simulink model "Evaluate_positioning_control_action"  (R2016b)
settings: Solver=ode1  StartTime=0.0  StopTime=pre_time  FixedStep=T_sample  MinStep=1e-4  RelTol=1e-3
undefined symbols (not defined in the file): A_f, Activator, B_f, C_f, D_f, filter_initial_condition, Integral_action, out_int, pre_time, x_0, x_start
libraries: qbmove_library x2, QB_pacer_lib x1
settings Model: Creator=Franco  LastModifiedBy=Franco
settings DataIOCC: LimitDataPoints=on  SaveFormat=Array  SignalLoggingSaveFormat=ModelDataLogs
settings OptimizationCC: ExpressionDepthLimit=2147483647  EfficientMapNaN2IntZero=off  LifeSpan=inf
settings DebuggingCC: UnderspecifiedInitializationDetection=Classic  MergeDetectMultiDrivingBlocksExec=none  SolverPrmCheckMsg=warning  FcnCallInpInsideContextMsg=warning  AllowSymbolicDim=off  StateNameClashWarn=warning  SFUnexpectedBacktrackingDiag=warning  SFNoUnconditionalDefaultTransitionDiag=warning  SFExecutionAtInitializationDiag=none
settings HardwareCC: ProdBitPerPointer=32  ProdBitPerSizeT=32  ProdBitPerPtrDiffT=32  ProdLargestAtomicFloat=None  ProdIntDivRoundTo=Undefined  ProdEndianess=Unspecified  ProdWordSize=32  ProdHWDeviceType=32-bit Generic  TargetBitPerPointer=64  TargetBitPerSizeT=64  TargetBitPerPtrDiffT=64  TargetLongLongMode=on  TargetIntDivRoundTo=Zero  TargetEndianess=LittleEndian  TargetWordSize=64  TargetHWDeviceType=MATLAB Host  ProdEqTarget=off
settings ModelReferenceCC: PropagateSignalLabelsOutOfModel=off
settings CodeAppCC: MaxIdLength=128
settings GRTTargetCC: TargetLangStandard=C89/C90 (ANSI)  GeneratePreprocessorConditionals=Disable all  CombineOutputUpdateFcns=off  GRTInterface=on
settings ConfigComp: CovMetricSettings=dw  CovHtmlReporting=on  CovSaveCumulativeToWorkspaceVar=on  CovSaveSingleToWorkspaceVar=on  CovExternalEMLEnable=off  CovSFcnEnable=off
settings ConfigurationSet: Description=SimMechanics 2G

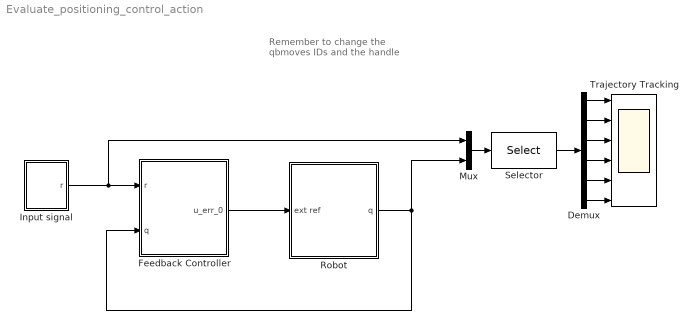
== system Evaluate_positioning_control_action ==
  note: Remember to change the qbmoves IDs and the handle
  Demux : Demux  Outputs=[2 2 2 2 2 2]
  Feedback Controller : Subsystem
  Input signal : Subsystem
  Mux : Mux  Inputs=2
  Robot : Subsystem
  Selector : Selector  InputPortWidth=12  IndexOptions=Index vector (dialog)  Indices=[1 7 2 8 3 9 4 10 5 11 6 12]  OutputSizes=1
  Trajectory Tracking : Scope  NumInputPorts=6
  wires:
  Feedback Controller/1(u_err_0) -> Robot/1("ext ref ")
  Robot/1(q) -> Feedback Controller/2(q), Mux/2
  Input signal/1(r) -> Mux/1, Feedback Controller/1(r)
  Mux/1 -> Selector/1
  Selector/1 -> Demux/1
  Demux/2 -> Trajectory Tracking/2
  Demux/3 -> Trajectory Tracking/3
  Demux/4 -> Trajectory Tracking/4
  Demux/5 -> Trajectory Tracking/5
  Demux/6 -> Trajectory Tracking/6
  Demux/1 -> Trajectory Tracking/1

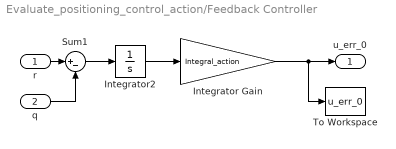
== system Evaluate_positioning_control_action/Feedback Controller ==
  r : Inport
  q : Inport  Port=2
  Integrator Gain : Gain  Gain=Integral_action
  Integrator2 : Integrator  InitialCondition=out_int
  Sum1 : Sum  Inputs=|+-
  To Workspace : ToWorkspace  VariableName=u_err_0  SaveFormat=Structure With Time  SampleTime=-1
  u_err_0 : Outport
  wires:
  r/1 -> Sum1/1
  q/1 -> Sum1/2
  Sum1/1 -> Integrator2/1
  Integrator2/1 -> Integrator Gain/1
  Integrator Gain/1 -> u_err_0/1, To Workspace/1

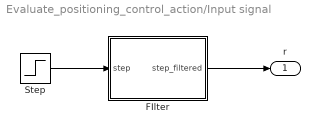
== system Evaluate_positioning_control_action/Input signal ==
  FIlter : Subsystem
  Step : Step  Time=pre_time/4  Before=x_start  After=x_0  SampleTime=0
  r : Outport
  wires:
  Step/1 -> FIlter/1(step)
  FIlter/1(step_filtered) -> r/1

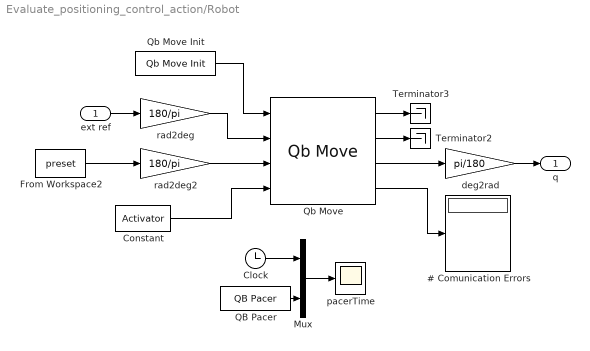
== system Evaluate_positioning_control_action/Robot ==
  "ext ref " : Inport
  # Comunication Errors : Display
  Clock : Clock
  Constant : Constant  Value=Activator
  From Workspace2 : FromWorkspace  VariableName=preset  SampleTime=0  OutputAfterFinalValue=Setting to zero
  Mux : Mux  Inputs=2
  QB Pacer : QB_pacer_lib/QB Pacer  simTimePerRealTime=1
  Qb Move : qbmove_library/Qb Move  ID=[1 2 3 4 5 6]  ACTIVE_COMM_DIRECTIONS=Both  CONTROL_MODE=Equilibrium Position and Stiffness Preset  DAISY_CHAINING=off  MAX_ANG=0  SW_LIMIT=inf  OFFSET=0  ACTIVATE=off  WDT=0.0  UNIT=Degrees
  Qb Move Init : qbmove_library/Qb Move Init  NUMBER_OF_COM='COM7'  BAUD_RATE_COM=2000000
  Terminator2 : Terminator
  Terminator3 : Terminator
  deg2rad : Gain  Gain=pi/180
  pacerTime : Scope
  rad2deg : Gain  Gain=180/pi
  rad2deg2 : Gain  Gain=180/pi
  q : Outport
  wires:
  deg2rad/1 -> q/1
  "ext ref "/1 -> rad2deg/1
  From Workspace2/1 -> rad2deg2/1
  QB Pacer/1 -> Mux/2
  Clock/1 -> Mux/1
  Qb Move Init/1 -> Qb Move/1
  Mux/1 -> pacerTime/1
  Qb Move/1 -> Terminator3/1
  Qb Move/2 -> Terminator2/1
  Qb Move/3 -> deg2rad/1
  rad2deg/1 -> Qb Move/2
  Qb Move/4 -> # Comunication Errors/1
  rad2deg2/1 -> Qb Move/3
  Constant/1 -> Qb Move/4

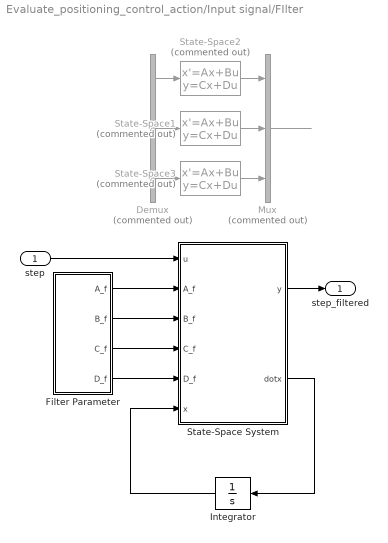
== system Evaluate_positioning_control_action/Input signal/FIlter ==
  step : Inport
  Demux : Demux  Commented=on  Outputs=3
  Filter Parameter : Subsystem
  Integrator : Integrator  InitialCondition=filter_initial_condition
  Mux : Mux  Commented=on  Inputs=3
  State-Space System : MATLAB Function  TreatAsAtomicUnit=on
  State-Space1 : StateSpace  Commented=on  A=A_f  B=B_f  C=C_f  D=D_f  X0=x_start(2)/C_f
  State-Space2 : StateSpace  Commented=on  A=A_f  B=B_f  C=C_f  D=D_f  X0=x_start(1)/C_f
  State-Space3 : StateSpace  Commented=on  A=A_f  B=B_f  C=C_f  D=D_f  X0=x_start(3)/C_f
  step_filtered : Outport
  wires:
  Demux/2 -> State-Space1/1
  Demux/3 -> State-Space3/1
  State-Space3/1 -> Mux/3
  State-Space1/1 -> Mux/2
  State-Space2/1 -> Mux/1
  Demux/1 -> State-Space2/1
  Mux/1 -> ?
  step/1 -> State-Space System/1(u)
  Filter Parameter/2(B_f) -> State-Space System/3(B_f)
  Filter Parameter/3(C_f) -> State-Space System/4(C_f)
  State-Space System/2(dotx) -> Integrator/1
  Filter Parameter/4(D_f) -> State-Space System/5(D_f)
  Integrator/1 -> State-Space System/6(x)
  Filter Parameter/1(A_f) -> State-Space System/2(A_f)
  State-Space System/1(y) -> step_filtered/1

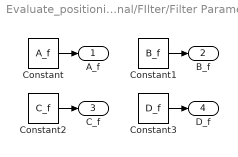
== system Evaluate_positioning_control_action/Input signal/FIlter/Filter Parameter ==
  Constant : Constant  Value=A_f
  Constant1 : Constant  Value=B_f
  Constant2 : Constant  Value=C_f
  Constant3 : Constant  Value=D_f
  A_f : Outport
  B_f : Outport  Port=2
  C_f : Outport  Port=3
  D_f : Outport  Port=4
  wires:
  Constant3/1 -> D_f/1
  Constant/1 -> A_f/1
  Constant1/1 -> B_f/1
  Constant2/1 -> C_f/1

== matlab function Evaluate_positioning_control_action/Input signal/FIlter/State-Space System ==
  data: u input; A_f input; B_f input; C_f input; D_f input; y output; x input; dotx output
%% Filter the input step signal with ss(A_f,B_f,C_f,D_f)
% Both number of joints and filter dimensions can vary
function [y,dotx] = fcn(u, A_f,B_f,C_f,D_f, x)
    [size_u,~] = size(u);
    [size_A,~] = size(A_f);
    
    res1 = zeros(size_A*size_u,1);
    res2 = zeros(size_u,1);
    
    for i = 1:size_u
       res1((i-1)*size_A + 1: i*size_A) =  A_f*x((i-1)*size_A + 1: i*size_A) + B_f*u(i);
       res2(i) = C_f'*x((i-1)*size_A + 1: i*size_A)+D_f*u(i);
    end 

    dotx = res1;
    y = res2;
end
